simulink model "bh_rolling_wheel_sim"  (R2022b)
settings: Solver=ode45  StartTime=0.0  StopTime=25  RelTol=1e-8  AbsTol=1e-8  EnableMultiTasking=on
undefined symbols (not defined in the file or in its folder): params_T
settings Model: Creator=bhorton  LastModifiedBy=bhorton
settings SolverCC: ZeroCrossAlgorithm=Adaptive  AlgebraicLoopSolver=TrustRegion
settings DataIOCC: LimitDataPoints=on  MaxDataPoints=10000
settings OptimizationCC: LifeSpan=inf
settings DebuggingCC: UnconnectedInputMsg=warning  UnconnectedOutputMsg=warning  UnconnectedLineMsg=warning  AllowSymbolicDim=off  SFUnexpectedBacktrackingDiag=warning  SFNoUnconditionalDefaultTransitionDiag=warning  SFExecutionAtInitializationDiag=none  SFMachineParentedDataDiag=warning  ArithmeticOperatorsInVariantConditions=warning
settings ModelReferenceCC: EnableRefExpFcnMdlSchedulingChecks=on
settings SFSimCC: SimUseLocalCustomCode=off  CustomCodeUndefinedFunction=UseInterfaceOnly
settings RTWCC: RTWUseLocalCustomCode=off  DLArmComputeVersion=19.05
settings CodeAppCC: StateflowObjectComments=on
settings GRTTargetCC: TargetLangStandard=C89/C90 (ANSI)
settings ConfigComp: CovMetricSettings=dw  CovSaveCumulativeToWorkspaceVar=on  CovSaveSingleToWorkspaceVar=on  CovExternalEMLEnable=off  CovSFcnEnable=off
settings SimscapeCC: SimscapeLogType=all  SimscapeLogSimulationStatistics=on  SimscapeLogDataHistory=10000
settings ExplorerConfigSet: InternalSimMechanicsExplorerSettings="<ExplorerConfiguration><canonicalview>default</canonicalview><AnimationSetting><BasePlaybackSpeed>1.0</BasePlaybackSpeed><PlaybackSpeedFactor>1.0</PlaybackSpeedFactor></AnimationSetting><TilePanel><TileInfo><Tiles Columns=\"2\" Count=\"3\" Rows=\"2\"><Column Weight=\"0.5\"/><Column Weight=\"0.5\"/><Row Weight=\"0.4994\"/><Row Weight=\"0.5006\"/><Tile Height=\"2\" Width=\"1\" X=\"0\" Y=\"0\"/><Tile Height=\"1\" Width=\"1\" X=\"1\" Y=\"0\"/><Tile Height=\"1\" Width=\"1\" X=\"1\" Y=\"1\"/></Tiles></TileInfo><SceneInfo><SceneViewer><BGColor><R>0.60000002384185791</R><G>0.60000002384185791</G><B>0.60000002384185791</B></BGColor><Camera><DoPerspective>off</DoPerspective><Position><X>2.72907980115163751</X><Y>1.63827710737355892</Y><Z>5.84466597133086818</Z></Position><Center><X>1.48957165804863778</X><Y>-0.312477395456248752</Y><Z>2.71114995707715156</Z></Center><Up><X>0.0871556787867786148</X><Y>0.8298702872998307</Y><Z>-0.551107243567087735</Z></Up><ViewLimDist>1</ViewLimDist><YLim>4.64142070213328051</YLim><XLim>3.96508464876347011</XLim></Camera></SceneViewer><SceneViewer><BGColor><R>0.60000002384185791</R><G>0.60000002384185791</G><B>0.60000002384185791</B></BGColor><Camera><DoPerspective>off</DoPerspective><Position><X>-0.00896342860419406529</X><Y>2.79833015796241735</Y><Z>0.117073013098141165</Z></Position><Center><X>-0.00541187908644796822</X><Y>-0.924820445952873049</Y><Z>0.115633039008129823</Z></Center><Up><X>0.00583965905908712894</X><Y>0.000392326129121878253</Y><Z>-0.999982872084458463</Z></Up><ViewLimDist>1</ViewLimDist><YLim>1.79047863545517116</YLim><XLim>3.09704412619272862</XLim></Camera></SceneViewer><SceneViewer><BGColor><R>0.60000002384185791</R><G>0.60000002384185791</G><B>0.60000002384185791</B></BGColor><Camera><DoPerspective>off</DoPerspective><Position><X>-0.273643330341835023</X><Y>-1.00050075945724948</Y><Z>3.33959185103632006</Z></Position><Center><X>-0.273643330341835023</X><Y>-1.00050075945724948</Y><Z>-3.69061607941034708e-08</Z></Center><Up><X>0</X><Y>1</Y><Z>-0</Z></Up><ViewLimDist>1</ViewLimDist><YLim>2.44671875206990475</YLim><XLim>4.21318386006656276</XLim></Camera></SceneViewer></SceneInfo></TilePanel><MechEditorPanel><Cameras/><GfxPanelCameraMap/><VideoCreator><PlaybackSpeedRatio>1.0</PlaybackSpeedRatio><FrameRate>30</FrameRate><VideoFormat>Motion JPEG AVI</VideoFormat><FrameSize>auto</FrameSize></VideoCreator></MechEditorPanel></ExplorerConfiguration>"

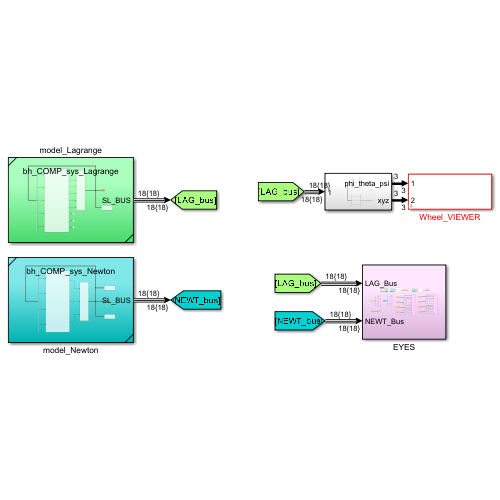
[thumbnail: Simulink's stored preview of the top-level diagram]
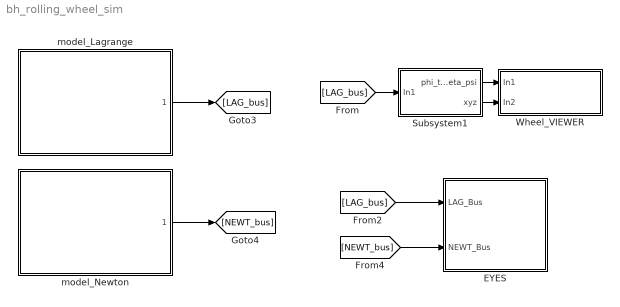
== system bh_rolling_wheel_sim ==
  EYES : Subsystem
  Subsystem1 : Subsystem
  Wheel_VIEWER : Subsystem  mask{Ts=0.01, R=params_T.r, the_XLIM=[-1,4], the_YLIM=[-2,3], yn_create_gif=off}
      mask prompts: Ts "Sample Time"; R "Wheel radius (m)"; the_XLIM "X axis display limita"; the_YLIM "Y axis display limita"; yn_create_gif "Create a Gif animation"
      mask init:
      | tf_create_gif = false;
      | 
      | if(1 == yn_create_gif)
      |     tf_create_gif = true;
      | end
  model_Lagrange : Subsystem  ReferencedSubsystem=bh_COMP_sys_Lagrange
  model_Newton : Subsystem  ReferencedSubsystem=bh_COMP_sys_Newton
  wires:
  model_Lagrange/1 -> [LAG_bus]
  [LAG_bus] -> EYES/1(LAG_Bus)
  model_Newton/1 -> [NEWT_bus]
  [NEWT_bus] -> EYES/2(NEWT_Bus)
  [LAG_bus] -> Subsystem1/1(In1)
  Subsystem1/1(phi_theta_psi) -> Wheel_VIEWER/1(In1)
  Subsystem1/2(xyz) -> Wheel_VIEWER/2(In2)

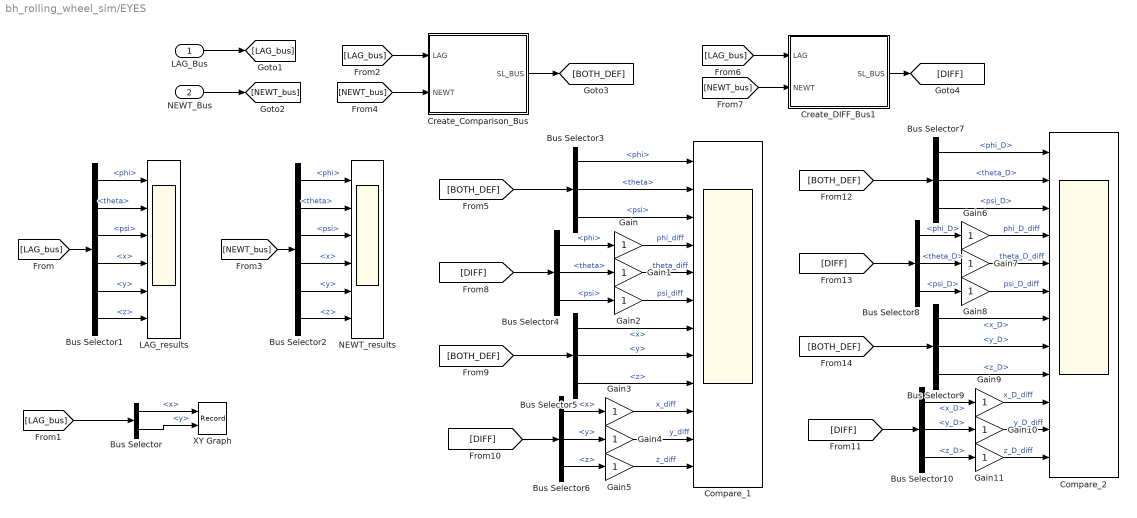
== system bh_rolling_wheel_sim/EYES ==
  LAG_Bus : Inport
  NEWT_Bus : Inport  Port=2
  Bus Selector : BusSelector  OutputSignals=x,y
  Bus Selector1 : BusSelector  OutputSignals=phi,theta,psi,x,y,z
  Bus Selector10 : BusSelector  OutputSignals=x_D,y_D,z_D
  Bus Selector2 : BusSelector  OutputSignals=phi,theta,psi,x,y,z
  Bus Selector3 : BusSelector  OutputSignals=phi,theta,psi
  Bus Selector4 : BusSelector  OutputSignals=phi,theta,psi
  Bus Selector5 : BusSelector  OutputSignals=x,y,z
  Bus Selector6 : BusSelector  OutputSignals=x,y,z
  Bus Selector7 : BusSelector  OutputSignals=phi_D,theta_D,psi_D
  Bus Selector8 : BusSelector  OutputSignals=phi_D,theta_D,psi_D
  Bus Selector9 : BusSelector  OutputSignals=x_D,y_D,z_D
  Compare_1 : Scope  NumInputPorts=12
  Compare_2 : Scope  NumInputPorts=12
  Create_Comparison_Bus : Subsystem
  Create_DIFF_Bus1 : Subsystem
  Gain{,1..11} (12 alike) : Gain
  LAG_results : Scope  NumInputPorts=6
  NEWT_results : Scope  NumInputPorts=6
  XY Graph : Record  FileSettingsInternal="{\"entries\":[{\"content\":{\"excelSettings\":{\"content\":{},\"type\":\"Streamout.ExcelSettings\"}},\"type\":\"Streamout.FileSettingStorage\",\"uuid\":\"3bbcc6d4-e80f-4088-86fa-dfbbbb3db5ed\"}],\"packageUris\":[\"http://schema.mathworks.com/mf0/streamout_blocks/R2020a\"],\"version\":\"1.0\"}"  Layout=[1 1]  SignalsInternal="{\"entries\":[{\"content\":{\"signals\":[{\"content\":{\"blockPath\":[\"bh_rolling_wheel_sim/EYES/XY Graph\"],\"channel\":[],\"dimensions\":[1],\"domain\":\"bh_rolling_wheel_sim/EYES/XY Graph\",\"lineColor\":\"#a2142f\",\"plots\":[1],\"port\":1,\"sid\":[\"\"],\"signalID\":276,\"signalName\":\"<x>\"},\"type\":\"RecordBlkView.Signal\",\"uuid\":\"79d595cb-14e4-4e82-960c-d63856479ab5\"},{\"content\":{\"blockPath\":[\"bh_rolling_wheel_sim/EYES/XY Graph\"],\"channel\":[],\"dimensions\":[1],\"domain\":\"bh_rolling_wheel_sim/EYES/XY Graph\",\"lineColor\":\"#139fff\",\"plots\":[1],\"port\":2,\"sid\":[\"\"],\"signalID\":280,\"signalName\":\"<y>\"},\"type\":\"RecordBlkView.Signal\",\"uuid\":\"96d2b0eb-df74-46b9-8e88-be5965efdb28\"}]},\"type\":\"RecordBlkView.InputSignals\",\"uuid\":\"0337ab20-17b4-4a58-be16-674d9728b6b7\"}],\"packageUris\":[\"http://schema.mathworks.com/mf0/streamout_blocks/R2020a\"],\"version\":\"1.0\"}"  VisualizationBindings="{\"xyplotplugin\":{\"info\":[{\"series\":[{\"bindingParametersList\":[{\"parameter\":\"X-Axis\",\"signalID\":276,\"signalName\":\"<x>\"},{\"parameter\":\"Y-Axis\",\"signalID\":280,\"signalName\":\"<y>\"}],\"seriesID\":22220}],\"subplotID\":1}]}}"  CompatibilityTag=XY  st=-1
  wires:
  LAG_Bus/1 -> [LAG_bus]
  [LAG_bus] -> Bus Selector1/1
  Bus Selector1/1 -> LAG_results/1  "<phi>"
  Bus Selector1/2 -> LAG_results/2  "<theta>"
  Bus Selector1/3 -> LAG_results/3  "<psi>"
  Bus Selector1/4 -> LAG_results/4  "<x>"
  Bus Selector1/5 -> LAG_results/5  "<y>"
  Bus Selector1/6 -> LAG_results/6  "<z>"
  [LAG_bus] -> Bus Selector/1
  Bus Selector/1 -> XY Graph/1  "<x>"
  Bus Selector/2 -> XY Graph/2  "<y>"
  NEWT_Bus/1 -> [NEWT_bus]
  Bus Selector2/5 -> NEWT_results/5  "<y>"
  Bus Selector2/4 -> NEWT_results/4  "<x>"
  Bus Selector2/2 -> NEWT_results/2  "<theta>"
  Bus Selector2/1 -> NEWT_results/1  "<phi>"
  Bus Selector2/6 -> NEWT_results/6  "<z>"
  [NEWT_bus] -> Bus Selector2/1
  Bus Selector2/3 -> NEWT_results/3  "<psi>"
  Create_Comparison_Bus/1(SL_BUS) -> [BOTH_DEF]
  [NEWT_bus] -> Create_Comparison_Bus/2(NEWT)
  [LAG_bus] -> Create_Comparison_Bus/1(LAG)
  [NEWT_bus] -> Create_DIFF_Bus1/2(NEWT)
  [LAG_bus] -> Create_DIFF_Bus1/1(LAG)
  Create_DIFF_Bus1/1(SL_BUS) -> [DIFF]
  [BOTH_DEF] -> Bus Selector3/1
  Bus Selector3/1 -> Compare_1/1  "<phi>"
  Bus Selector3/2 -> Compare_1/2  "<theta>"
  Bus Selector3/3 -> Compare_1/3  "<psi>"
  Bus Selector4/1 -> Gain/1  "<phi>"
  Bus Selector4/2 -> Gain1/1  "<theta>"
  Bus Selector4/3 -> Gain2/1  "<psi>"
  [DIFF] -> Bus Selector4/1
  [BOTH_DEF] -> Bus Selector5/1
  Bus Selector5/1 -> Compare_1/7  "<x>"
  Bus Selector5/2 -> Compare_1/8  "<y>"
  Bus Selector5/3 -> Compare_1/9  "<z>"
  Bus Selector6/2 -> Gain4/1  "<y>"
  [DIFF] -> Bus Selector6/1
  Bus Selector6/1 -> Gain3/1  "<x>"
  Bus Selector6/3 -> Gain5/1  "<z>"
  Bus Selector9/1 -> Compare_2/7  "<x_D>"
  [BOTH_DEF] -> Bus Selector9/1
  Bus Selector9/3 -> Compare_2/9  "<z_D>"
  Bus Selector9/2 -> Compare_2/8  "<y_D>"
  Bus Selector7/1 -> Compare_2/1  "<phi_D>"
  Bus Selector7/2 -> Compare_2/2  "<theta_D>"
  Bus Selector7/3 -> Compare_2/3  "<psi_D>"
  [DIFF] -> Bus Selector8/1
  [DIFF] -> Bus Selector10/1
  [BOTH_DEF] -> Bus Selector7/1
  Gain2/1 -> Compare_1/6  "psi_diff"
  Gain/1 -> Compare_1/4  "phi_diff"
  Gain1/1 -> Compare_1/5  "theta_diff"
  Gain3/1 -> Compare_1/10  "x_diff"
  Gain4/1 -> Compare_1/11  "y_diff"
  Gain5/1 -> Compare_1/12  "z_diff"
  Bus Selector8/1 -> Gain6/1  "<phi_D>"
  Bus Selector8/2 -> Gain7/1  "<theta_D>"
  Bus Selector8/3 -> Gain8/1  "<psi_D>"
  Bus Selector10/1 -> Gain9/1  "<x_D>"
  Bus Selector10/2 -> Gain10/1  "<y_D>"
  Bus Selector10/3 -> Gain11/1  "<z_D>"
  Gain6/1 -> Compare_2/4  "phi_D_diff"
  Gain7/1 -> Compare_2/5  "theta_D_diff"
  Gain8/1 -> Compare_2/6  "psi_D_diff"
  Gain9/1 -> Compare_2/10  "x_D_diff"
  Gain10/1 -> Compare_2/11  "y_D_diff"
  Gain11/1 -> Compare_2/12  "z_D_diff"

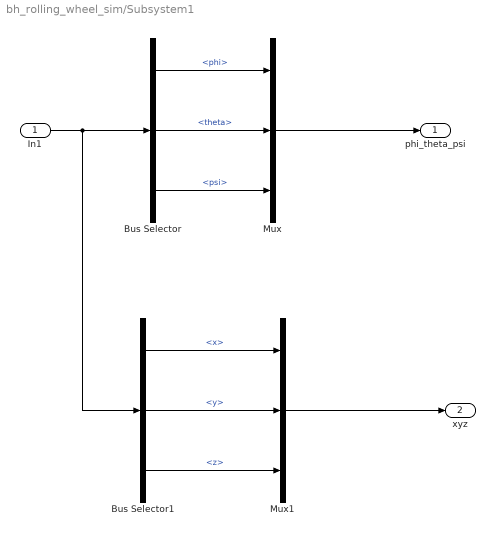
== system bh_rolling_wheel_sim/Subsystem1 ==
  In1 : Inport
  Bus Selector : BusSelector  OutputSignals=phi,theta,psi
  Bus Selector1 : BusSelector  OutputSignals=x,y,z
  Mux : Mux  Inputs=3
  Mux1 : Mux  Inputs=3
  phi_theta_psi : Outport
  xyz : Outport  Port=2
  wires:
  In1/1 -> Bus Selector1/1, Bus Selector/1
  Bus Selector/1 -> Mux/1  "<phi>"
  Bus Selector/2 -> Mux/2  "<theta>"
  Bus Selector/3 -> Mux/3  "<psi>"
  Bus Selector1/1 -> Mux1/1  "<x>"
  Bus Selector1/2 -> Mux1/2  "<y>"
  Bus Selector1/3 -> Mux1/3  "<z>"
  Mux/1 -> phi_theta_psi/1
  Mux1/1 -> xyz/1

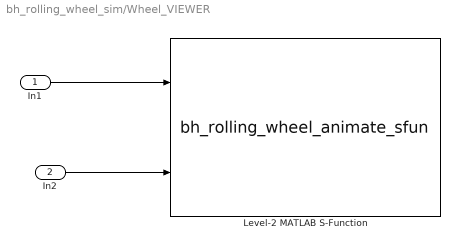
== system bh_rolling_wheel_sim/Wheel_VIEWER ==
  In1 : Inport
  In2 : Inport  Port=2
  Level-2 MATLAB S-Function : M-S-Function  FunctionName=bh_rolling_wheel_animate_sfun  Parameters=Ts, R, the_XLIM, the_YLIM, tf_create_gif
  wires:
  In1/1 -> Level-2 MATLAB S-Function/1
  In2/1 -> Level-2 MATLAB S-Function/2

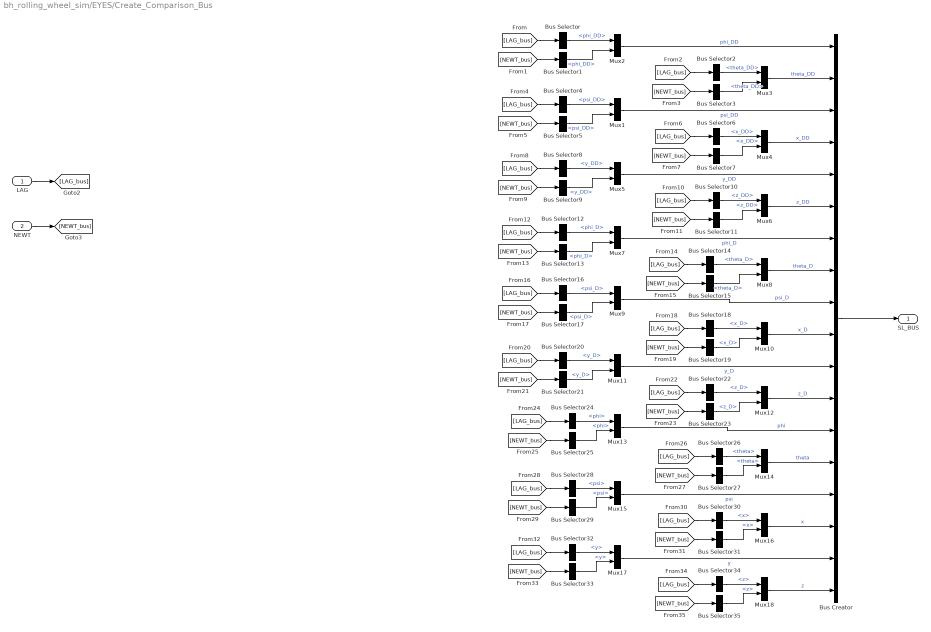
== system bh_rolling_wheel_sim/EYES/Create_Comparison_Bus ==
  LAG : Inport
  NEWT : Inport  Port=2
  Bus Creator : BusCreator  Inputs=18
  Bus Selector : BusSelector  OutputSignals=phi_DD
  Bus Selector1 : BusSelector  OutputSignals=phi_DD
  Bus Selector10 : BusSelector  OutputSignals=z_DD
  Bus Selector11 : BusSelector  OutputSignals=z_DD
  Bus Selector12 : BusSelector  OutputSignals=phi_D
  Bus Selector13 : BusSelector  OutputSignals=phi_D
  Bus Selector14 : BusSelector  OutputSignals=theta_D
  Bus Selector15 : BusSelector  OutputSignals=theta_D
  Bus Selector16 : BusSelector  OutputSignals=psi_D
  Bus Selector17 : BusSelector  OutputSignals=psi_D
  Bus Selector18 : BusSelector  OutputSignals=x_D
  Bus Selector19 : BusSelector  OutputSignals=x_D
  Bus Selector2 : BusSelector  OutputSignals=theta_DD
  Bus Selector20 : BusSelector  OutputSignals=y_D
  Bus Selector21 : BusSelector  OutputSignals=y_D
  Bus Selector22 : BusSelector  OutputSignals=z_D
  Bus Selector23 : BusSelector  OutputSignals=z_D
  Bus Selector24 : BusSelector  OutputSignals=phi
  Bus Selector25 : BusSelector  OutputSignals=phi
  Bus Selector26 : BusSelector  OutputSignals=theta
  Bus Selector27 : BusSelector  OutputSignals=theta
  Bus Selector28 : BusSelector  OutputSignals=psi
  Bus Selector29 : BusSelector  OutputSignals=psi
  Bus Selector3 : BusSelector  OutputSignals=theta_DD
  Bus Selector30 : BusSelector  OutputSignals=x
  Bus Selector31 : BusSelector  OutputSignals=x
  Bus Selector32 : BusSelector  OutputSignals=y
  Bus Selector33 : BusSelector  OutputSignals=y
  Bus Selector34 : BusSelector  OutputSignals=z
  Bus Selector35 : BusSelector  OutputSignals=z
  Bus Selector4 : BusSelector  OutputSignals=psi_DD
  Bus Selector5 : BusSelector  OutputSignals=psi_DD
  Bus Selector6 : BusSelector  OutputSignals=x_DD
  Bus Selector7 : BusSelector  OutputSignals=x_DD
  Bus Selector8 : BusSelector  OutputSignals=y_DD
  Bus Selector9 : BusSelector  OutputSignals=y_DD
  Mux{1..18} (18 alike) : Mux  Inputs=2
  SL_BUS : Outport
  wires:
  NEWT/1 -> [NEWT_bus]
  LAG/1 -> [LAG_bus]
  [LAG_bus] -> Bus Selector/1
  [NEWT_bus] -> Bus Selector1/1
  Bus Selector/1 -> Mux2/1  "<phi_DD>"
  Bus Selector1/1 -> Mux2/2  "<phi_DD>"
  Mux3/1 -> Bus Creator/2  "theta_DD"
  Mux13/1 -> Bus Creator/13  "phi"
  Mux18/1 -> Bus Creator/18  "z"
  Mux16/1 -> Bus Creator/16  "x"
  Mux15/1 -> Bus Creator/15  "psi"
  Mux9/1 -> Bus Creator/9  "psi_D"
  Mux8/1 -> Bus Creator/8  "theta_D"
  Mux12/1 -> Bus Creator/12  "z_D"
  Mux11/1 -> Bus Creator/11  "y_D"
  Mux17/1 -> Bus Creator/17  "y"
  Mux5/1 -> Bus Creator/5  "y_DD"
  Mux14/1 -> Bus Creator/14  "theta"
  Bus Creator/1 -> SL_BUS/1
  Mux7/1 -> Bus Creator/7  "phi_D"
  Mux10/1 -> Bus Creator/10  "x_D"
  Mux6/1 -> Bus Creator/6  "z_DD"
  Mux4/1 -> Bus Creator/4  "x_DD"
  Mux1/1 -> Bus Creator/3  "psi_DD"
  Mux2/1 -> Bus Creator/1  "phi_DD"
  [LAG_bus] -> Bus Selector2/1
  [NEWT_bus] -> Bus Selector3/1
  Bus Selector2/1 -> Mux3/1  "<theta_DD>"
  Bus Selector3/1 -> Mux3/2  "<theta_DD>"
  Bus Selector5/1 -> Mux1/2  "<psi_DD>"
  [LAG_bus] -> Bus Selector4/1
  Bus Selector4/1 -> Mux1/1  "<psi_DD>"
  [NEWT_bus] -> Bus Selector5/1
  Bus Selector6/1 -> Mux4/1  "<x_DD>"
  [NEWT_bus] -> Bus Selector7/1
  [LAG_bus] -> Bus Selector6/1
  Bus Selector7/1 -> Mux4/2  "<x_DD>"
  Bus Selector8/1 -> Mux5/1  "<y_DD>"
  [LAG_bus] -> Bus Selector8/1
  [NEWT_bus] -> Bus Selector9/1
  Bus Selector9/1 -> Mux5/2  "<y_DD>"
  Bus Selector10/1 -> Mux6/1  "<z_DD>"
  Bus Selector11/1 -> Mux6/2  "<z_DD>"
  [LAG_bus] -> Bus Selector10/1
  [NEWT_bus] -> Bus Selector11/1
  Bus Selector13/1 -> Mux7/2  "<phi_D>"
  [LAG_bus] -> Bus Selector12/1
  Bus Selector12/1 -> Mux7/1  "<phi_D>"
  [NEWT_bus] -> Bus Selector13/1
  Bus Selector14/1 -> Mux8/1  "<theta_D>"
  [NEWT_bus] -> Bus Selector15/1
  [LAG_bus] -> Bus Selector14/1
  Bus Selector15/1 -> Mux8/2  "<theta_D>"
  [NEWT_bus] -> Bus Selector17/1
  [LAG_bus] -> Bus Selector16/1
  Bus Selector17/1 -> Mux9/2  "<psi_D>"
  Bus Selector16/1 -> Mux9/1  "<psi_D>"
  Bus Selector19/1 -> Mux10/2  "<x_D>"
  [LAG_bus] -> Bus Selector18/1
  Bus Selector18/1 -> Mux10/1  "<x_D>"
  [NEWT_bus] -> Bus Selector19/1
  Bus Selector20/1 -> Mux11/1  "<y_D>"
  [LAG_bus] -> Bus Selector20/1
  [NEWT_bus] -> Bus Selector21/1
  Bus Selector21/1 -> Mux11/2  "<y_D>"
  [NEWT_bus] -> Bus Selector23/1
  Bus Selector23/1 -> Mux12/2  "<z_D>"
  [LAG_bus] -> Bus Selector22/1
  Bus Selector22/1 -> Mux12/1  "<z_D>"
  [NEWT_bus] -> Bus Selector25/1
  [LAG_bus] -> Bus Selector24/1
  Bus Selector24/1 -> Mux13/1  "<phi>"
  Bus Selector25/1 -> Mux13/2  "<phi>"
  [LAG_bus] -> Bus Selector26/1
  [NEWT_bus] -> Bus Selector27/1
  Bus Selector27/1 -> Mux14/2  "<theta>"
  Bus Selector26/1 -> Mux14/1  "<theta>"
  Bus Selector29/1 -> Mux15/2  "<psi>"
  Bus Selector28/1 -> Mux15/1  "<psi>"
  [LAG_bus] -> Bus Selector28/1
  [NEWT_bus] -> Bus Selector29/1
  Bus Selector31/1 -> Mux16/2  "<x>"
  Bus Selector30/1 -> Mux16/1  "<x>"
  [LAG_bus] -> Bus Selector30/1
  [NEWT_bus] -> Bus Selector31/1
  [NEWT_bus] -> Bus Selector33/1
  [LAG_bus] -> Bus Selector32/1
  Bus Selector32/1 -> Mux17/1  "<y>"
  Bus Selector33/1 -> Mux17/2  "<y>"
  [NEWT_bus] -> Bus Selector35/1
  Bus Selector35/1 -> Mux18/2  "<z>"
  [LAG_bus] -> Bus Selector34/1
  Bus Selector34/1 -> Mux18/1  "<z>"

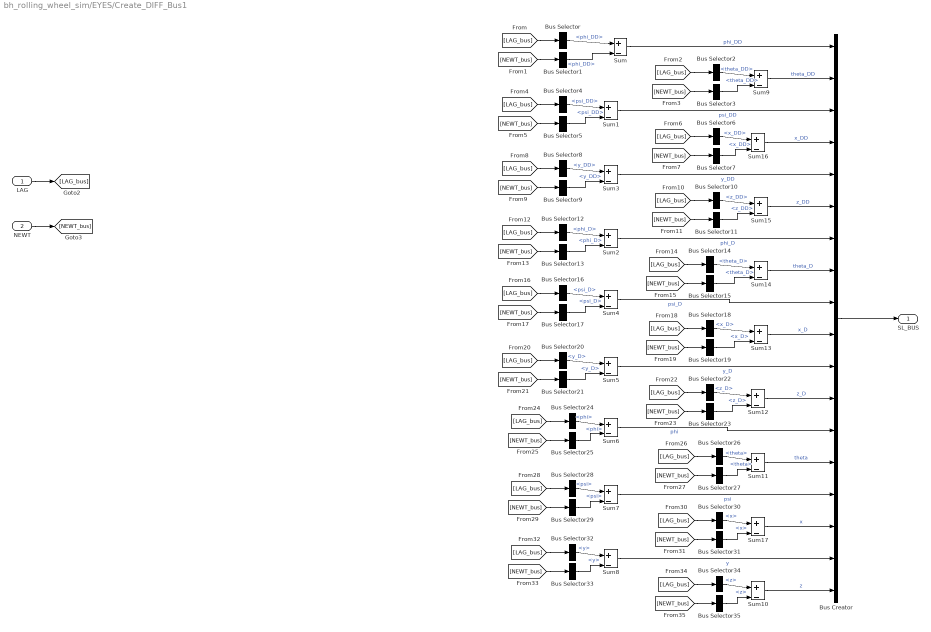
== system bh_rolling_wheel_sim/EYES/Create_DIFF_Bus1 ==
  LAG : Inport
  NEWT : Inport  Port=2
  Bus Creator : BusCreator  Inputs=18
  Bus Selector : BusSelector  OutputSignals=phi_DD
  Bus Selector1 : BusSelector  OutputSignals=phi_DD
  Bus Selector10 : BusSelector  OutputSignals=z_DD
  Bus Selector11 : BusSelector  OutputSignals=z_DD
  Bus Selector12 : BusSelector  OutputSignals=phi_D
  Bus Selector13 : BusSelector  OutputSignals=phi_D
  Bus Selector14 : BusSelector  OutputSignals=theta_D
  Bus Selector15 : BusSelector  OutputSignals=theta_D
  Bus Selector16 : BusSelector  OutputSignals=psi_D
  Bus Selector17 : BusSelector  OutputSignals=psi_D
  Bus Selector18 : BusSelector  OutputSignals=x_D
  Bus Selector19 : BusSelector  OutputSignals=x_D
  Bus Selector2 : BusSelector  OutputSignals=theta_DD
  Bus Selector20 : BusSelector  OutputSignals=y_D
  Bus Selector21 : BusSelector  OutputSignals=y_D
  Bus Selector22 : BusSelector  OutputSignals=z_D
  Bus Selector23 : BusSelector  OutputSignals=z_D
  Bus Selector24 : BusSelector  OutputSignals=phi
  Bus Selector25 : BusSelector  OutputSignals=phi
  Bus Selector26 : BusSelector  OutputSignals=theta
  Bus Selector27 : BusSelector  OutputSignals=theta
  Bus Selector28 : BusSelector  OutputSignals=psi
  Bus Selector29 : BusSelector  OutputSignals=psi
  Bus Selector3 : BusSelector  OutputSignals=theta_DD
  Bus Selector30 : BusSelector  OutputSignals=x
  Bus Selector31 : BusSelector  OutputSignals=x
  Bus Selector32 : BusSelector  OutputSignals=y
  Bus Selector33 : BusSelector  OutputSignals=y
  Bus Selector34 : BusSelector  OutputSignals=z
  Bus Selector35 : BusSelector  OutputSignals=z
  Bus Selector4 : BusSelector  OutputSignals=psi_DD
  Bus Selector5 : BusSelector  OutputSignals=psi_DD
  Bus Selector6 : BusSelector  OutputSignals=x_DD
  Bus Selector7 : BusSelector  OutputSignals=x_DD
  Bus Selector8 : BusSelector  OutputSignals=y_DD
  Bus Selector9 : BusSelector  OutputSignals=y_DD
  Sum{,1..17} (18 alike) : Sum  Inputs=+|-
  SL_BUS : Outport
  wires:
  NEWT/1 -> [NEWT_bus]
  LAG/1 -> [LAG_bus]
  [LAG_bus] -> Bus Selector/1
  [NEWT_bus] -> Bus Selector1/1
  Bus Selector/1 -> Sum/1  "<phi_DD>"
  Bus Selector1/1 -> Sum/2  "<phi_DD>"
  Sum9/1 -> Bus Creator/2  "theta_DD"
  Sum6/1 -> Bus Creator/13  "phi"
  Sum10/1 -> Bus Creator/18  "z"
  Sum17/1 -> Bus Creator/16  "x"
  Sum7/1 -> Bus Creator/15  "psi"
  Sum4/1 -> Bus Creator/9  "psi_D"
  Sum14/1 -> Bus Creator/8  "theta_D"
  Sum12/1 -> Bus Creator/12  "z_D"
  Sum5/1 -> Bus Creator/11  "y_D"
  Sum8/1 -> Bus Creator/17  "y"
  Sum3/1 -> Bus Creator/5  "y_DD"
  Sum11/1 -> Bus Creator/14  "theta"
  Bus Creator/1 -> SL_BUS/1
  Sum2/1 -> Bus Creator/7  "phi_D"
  Sum13/1 -> Bus Creator/10  "x_D"
  Sum15/1 -> Bus Creator/6  "z_DD"
  Sum16/1 -> Bus Creator/4  "x_DD"
  Sum1/1 -> Bus Creator/3  "psi_DD"
  Sum/1 -> Bus Creator/1  "phi_DD"
  [LAG_bus] -> Bus Selector2/1
  [NEWT_bus] -> Bus Selector3/1
  Bus Selector2/1 -> Sum9/1  "<theta_DD>"
  Bus Selector3/1 -> Sum9/2  "<theta_DD>"
  [LAG_bus] -> Bus Selector4/1
  [NEWT_bus] -> Bus Selector5/1
  [NEWT_bus] -> Bus Selector7/1
  [LAG_bus] -> Bus Selector6/1
  [LAG_bus] -> Bus Selector8/1
  [NEWT_bus] -> Bus Selector9/1
  [LAG_bus] -> Bus Selector10/1
  [NEWT_bus] -> Bus Selector11/1
  [LAG_bus] -> Bus Selector12/1
  [NEWT_bus] -> Bus Selector13/1
  [NEWT_bus] -> Bus Selector15/1
  [LAG_bus] -> Bus Selector14/1
  [NEWT_bus] -> Bus Selector17/1
  [LAG_bus] -> Bus Selector16/1
  [LAG_bus] -> Bus Selector18/1
  [NEWT_bus] -> Bus Selector19/1
  [LAG_bus] -> Bus Selector20/1
  [NEWT_bus] -> Bus Selector21/1
  [NEWT_bus] -> Bus Selector23/1
  [LAG_bus] -> Bus Selector22/1
  [NEWT_bus] -> Bus Selector25/1
  [LAG_bus] -> Bus Selector24/1
  [LAG_bus] -> Bus Selector26/1
  [NEWT_bus] -> Bus Selector27/1
  [LAG_bus] -> Bus Selector28/1
  [NEWT_bus] -> Bus Selector29/1
  [LAG_bus] -> Bus Selector30/1
  [NEWT_bus] -> Bus Selector31/1
  [NEWT_bus] -> Bus Selector33/1
  [LAG_bus] -> Bus Selector32/1
  [NEWT_bus] -> Bus Selector35/1
  [LAG_bus] -> Bus Selector34/1
  Bus Selector4/1 -> Sum1/1  "<psi_DD>"
  Bus Selector5/1 -> Sum1/2  "<psi_DD>"
  Bus Selector8/1 -> Sum3/1  "<y_DD>"
  Bus Selector9/1 -> Sum3/2  "<y_DD>"
  Bus Selector12/1 -> Sum2/1  "<phi_D>"
  Bus Selector13/1 -> Sum2/2  "<phi_D>"
  Bus Selector16/1 -> Sum4/1  "<psi_D>"
  Bus Selector17/1 -> Sum4/2  "<psi_D>"
  Bus Selector20/1 -> Sum5/1  "<y_D>"
  Bus Selector21/1 -> Sum5/2  "<y_D>"
  Bus Selector24/1 -> Sum6/1  "<phi>"
  Bus Selector25/1 -> Sum6/2  "<phi>"
  Bus Selector28/1 -> Sum7/1  "<psi>"
  Bus Selector29/1 -> Sum7/2  "<psi>"
  Bus Selector32/1 -> Sum8/1  "<y>"
  Bus Selector33/1 -> Sum8/2  "<y>"
  Bus Selector6/1 -> Sum16/1  "<x_DD>"
  Bus Selector7/1 -> Sum16/2  "<x_DD>"
  Bus Selector10/1 -> Sum15/1  "<z_DD>"
  Bus Selector11/1 -> Sum15/2  "<z_DD>"
  Bus Selector14/1 -> Sum14/1  "<theta_D>"
  Bus Selector15/1 -> Sum14/2  "<theta_D>"
  Bus Selector18/1 -> Sum13/1  "<x_D>"
  Bus Selector19/1 -> Sum13/2  "<x_D>"
  Bus Selector22/1 -> Sum12/1  "<z_D>"
  Bus Selector23/1 -> Sum12/2  "<z_D>"
  Bus Selector26/1 -> Sum11/1  "<theta>"
  Bus Selector27/1 -> Sum11/2  "<theta>"
  Bus Selector30/1 -> Sum17/1  "<x>"
  Bus Selector31/1 -> Sum17/2  "<x>"
  Bus Selector34/1 -> Sum10/1  "<z>"
  Bus Selector35/1 -> Sum10/2  "<z>"
